simulink model "FrameStructTest"  (R2022b)
settings: Solver=VariableStepAuto  StartTime=0.0  StopTime=0.01  RelTol=1e-3
model workspace (MAT data in the model file):
  f_s = Simulink.Parameter
  f_s.Value = 0.0001
  f_s.DataType = 'double'
  f_s.Complexity = 'real'
  f_s.Dimensions = [1 1]
libraries: simulink x24, hdlsllib x14, dspsigops x8, commdigbbndapm x3, dsphdlfiltering2 x2, commfilt2 x2, commdigbbndpm3 x2, commrandsrc3 x1
(part 1 of 2)
settings Model: Creator=svdvl  LastModifiedBy=User

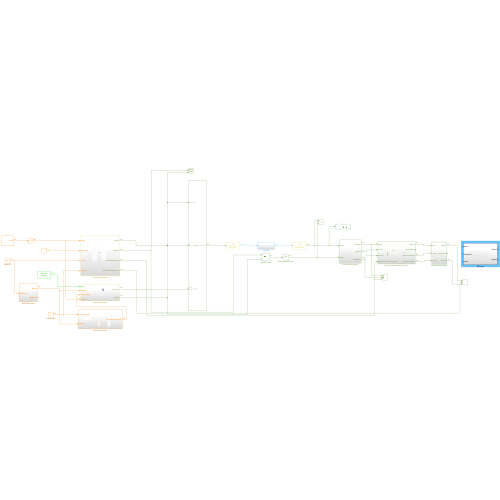
[thumbnail: Simulink's stored preview of the top-level diagram]
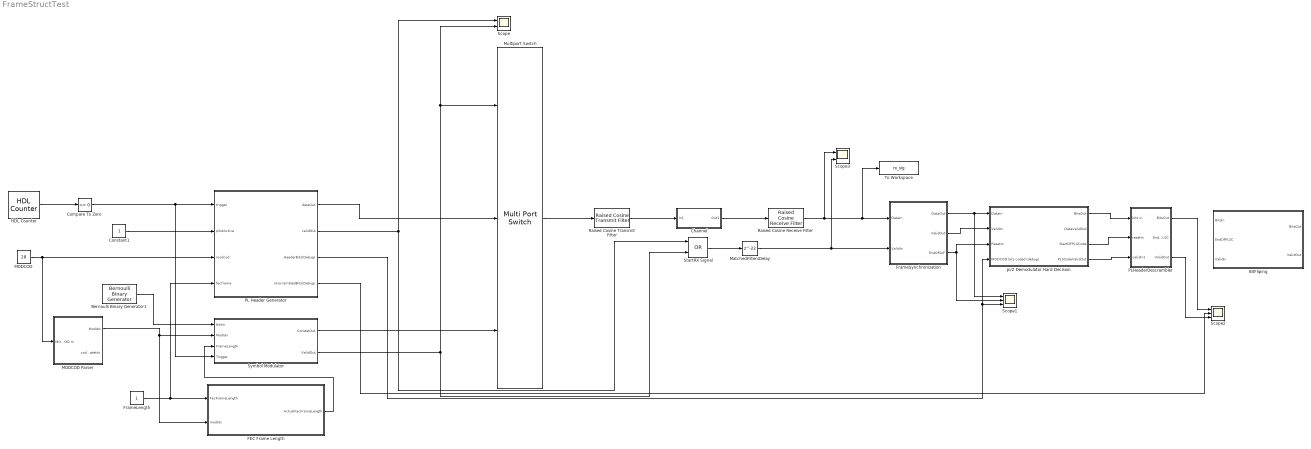
== system FrameStructTest ==
  Bernoulli Binary Generator1 : commrandsrc3/Bernoulli Binary Generator  ProbabilityOfZero=0.5  SeedSource=Auto  Seed=0  SampleTime=f_s/32*7/10  SamplesPerFrame=1  OutputDataType=uint8  SimulateUsing=Code generation
  BitFliping : Subsystem
  Channel : Subsystem
  Compare To Zero : simulink/Logic and Bit Operations/Compare To Zero  relop===  OutDataTypeStr=boolean
  Constant1 : Constant  SampleTime=f_s
  FEC Frame Length : Subsystem
  FrameLength : Constant  SampleTime=f_s
  FrameSynchronization : Subsystem
  HDL Counter : hdlsllib/Sources/HDL Counter  CountType=Count limited  CountInit=0  CountStep=1  CountMax=12960  CountFromType=Initial value  CountFrom=0  CountResetPort=off  CountLoadPort=off  CountEnbPort=off  CountDirPort=off  CountHitOutputPort=off  CountDataType=Unsigned  CountWordLen=14  CountFracLen=0  CountSampTime=f_s
  MODCOD : Constant  Value=28  VectorParams1D=off  OutDataTypeStr=uint8  SampleTime=f_s
  MODCOD Parser : Subsystem
  MatchedFiltersDelay : Delay  DelayLength=22
  Multiport Switch : MultiPortSwitch  DataPortOrder=Zero-based contiguous  Inputs=2  zeroidx=on  SaturateOnIntegerOverflow=off  InputSameDT=off
  PL Header Generator : Subsystem
  PLHeaderDescrambler : Subsystem
  Raised Cosine Receive Filter : commfilt2/Raised Cosine Receive Filter  filtType=Square root  R=0.2  filtSpan=20  N=2  downFactor=2  downOffset=0  filterGain=1  RateOptions=Allow multirate processing  framing=Mute  checkCoeff=off  variableName=rcRxFilt  currentFiltSpan=10  D=5  inputOffset=0  sampMode=Mute  saveAsFlag=0  rateMode=Downsampling  checkGain=Normalized  launchFVT=on  roundingMode=Floor  overflowMode=off  coeffDataTypeStr=Inherit: Same word length as input  coeffMin=[]  coeffMax=[]  coeffLastDataTypeStr=Inherit: Same word length as input  accumDataTypeStr=Inherit: Same as product output  accumLastDataTypeStr=Inherit: Same as product output  outputDataTypeStr=Inherit: Same as accumulator  outputMin=[]  outputMax=[]  outputLastDataTypeStr=Inherit: Same as accumulator
      settings: LibrarySourceBlock=|
      | commhdlfilt/Raised Cosine
      | Receive Filter
  Raised Cosine Transmit Filter : commfilt2/Raised Cosine Transmit Filter  filtType=Square root  R=0.2  filtSpan=20  N=2  filterGain=1  RateOptions=Allow multirate processing  framing=Mute  checkCoeff=off  variableName=rcTxFilt  checkGain=Normalized  sampMode=Mute  saveAsFlag=0  currentFiltSpan=10  D=5  launchFVT=on  roundingMode=Floor  overflowMode=off  coeffDataTypeStr=Inherit: Same word length as input  coeffMin=[]  coeffMax=[]  coeffLastDataTypeStr=Inherit: Same word length as input  outputDataTypeStr=Inherit: Same as accumulator  outputMin=[]  outputMax=[]  outputLastDataTypeStr=Inherit: Same as accumulator
      settings: LibrarySourceBlock=|
      | commhdlfilt/Raised Cosine
      | Transmit Filter
  Scope : Scope  NumInputPorts=2
  Scope1 : Scope  NumInputPorts=3
  Scope2 : Scope  NumInputPorts=3
  Scope3 : Scope  NumInputPorts=2
  StartRX Signal : Logic  Operator=OR  AllPortsSameDT=off  OutDataTypeStr=boolean
  Symbol Modulator : Subsystem
  To Workspace : ToWorkspace  VariableName=rx_sig  SampleTime=-1
      settings: Save2DSignal=2-D array (concatenate along first dimension)
  pi/2 Demodulator Hard Decision : Subsystem
  wires:
  HDL Counter/1 -> Compare To Zero/1
  FEC Frame Length/1(ActualFecFrameLength) -> Symbol Modulator/3(FrameLength)
  MODCOD Parser/1(ModIdx) -> FEC Frame Length/2(modIdx), Symbol Modulator/2(ModIdx)
  Bernoulli Binary Generator1/1 -> Symbol Modulator/1(bitsIn)
  Symbol Modulator/1(ConstelOut) -> Multiport Switch/3
  MODCOD/1 -> PL Header Generator/3(modcod), MODCOD Parser/1(MODCOD In)
  FrameLength/1 -> PL Header Generator/4(fecframe), FEC Frame Length/1(FecFrameLength)
  Compare To Zero/1 -> PL Header Generator/1(trigger), Symbol Modulator/4(Trigger)
  PL Header Generator/2(validOut) -> StartRX Signal/1, Scope/1
  Symbol Modulator/2(ValidOut) -> StartRX Signal/2, Multiport Switch/1, Scope/2
  PL Header Generator/1(dataOut) -> Multiport Switch/2
  Raised Cosine Transmit Filter/1 -> Channel/1(In1)
  Channel/1(Out1) -> Raised Cosine Receive Filter/1
  Raised Cosine Receive Filter/1 -> Scope3/1, To Workspace/1, FrameSynchronization/1(DataIn)
  Multiport Switch/1 -> Raised Cosine Transmit Filter/1
  FrameSynchronization/1(DataOut) -> Scope1/1, pi/2 Demodulator Hard Decision/1(DataIn)
  FrameSynchronization/2(ValidOut) -> pi/2 Demodulator Hard Decision/2(ValidIn)
  FrameSynchronization/3(EndOfSoF) -> Scope1/2, pi/2 Demodulator Hard Decision/3(ResetIn)
  PL Header Generator/3(HeaderBits(Debug)) -> Scope1/3, pi/2 Demodulator Hard Decision/4(MODCOD bits coded (debug))
  pi/2 Demodulator Hard Decision/1(BitsOut) -> PLHeaderDescrambler/1(bits in)
  pi/2 Demodulator Hard Decision/3(StartOFPLSCode) -> PLHeaderDescrambler/2(resetIn)
  pi/2 Demodulator Hard Decision/4(PLSCodeValidOut) -> PLHeaderDescrambler/3(validIn1)
  PLHeaderDescrambler/1(BitsOut) -> Scope2/1
  PL Header Generator/4(UnscrambledBits(Debug)) -> Scope2/2
  PLHeaderDescrambler/3(ValidOut) -> Scope2/3
  Constant1/1 -> PL Header Generator/2(pilotActive)
  StartRX Signal/1 -> MatchedFiltersDelay/1
  MatchedFiltersDelay/1 -> Scope3/2, FrameSynchronization/2(ValidIn)

== system FrameStructTest/BitFliping ==
  note: Bit 7 at the output
  BitsIn : Inport
  EndOfPLSC : Inport  Port=2
  ValidIn : Inport  Port=3
  Delay : Delay  DelayLength=1
  Delay1 : Delay  DelayLength=1
  Enabled Delay : Delay  DelayLength=1  ShowEnablePort=on
      settings: InputPortMap=u0,e6
  HDL Counter : hdlsllib/Sources/HDL Counter  CountType=Count limited  CountInit=0  CountStep=1  CountMax=1  CountFromType=Initial value  CountFrom=0  CountResetPort=off  CountLoadPort=off  CountEnbPort=on  CountDirPort=off  CountHitOutputPort=off  CountDataType=Unsigned  CountWordLen=8  CountFracLen=0  CountSampTime=1
  Logical Operator : Logic  Operator=XOR  AllPortsSameDT=off  OutDataTypeStr=boolean
  Logical Operator1 : Logic  Operator=NOT  AllPortsSameDT=off  OutDataTypeStr=boolean
  Switch : Switch  Criteria=u2 > Threshold  SaturateOnIntegerOverflow=off  InputSameDT=off
  Switch1 : Switch  Criteria=u2 ~= 0  SaturateOnIntegerOverflow=off  InputSameDT=off
  BitsOut : Outport
  ValidOut : Outport  Port=2
  wires:
  BitsIn/1 -> Delay/1, Logical Operator1/1, Delay1/1, Switch/1, Logical Operator/1
  Delay/1 -> Logical Operator/2
  Switch1/1 -> BitsOut/1
  ValidIn/1 -> HDL Counter/1
  HDL Counter/1 -> Enabled Delay/2, Switch/2
  Logical Operator/1 -> Enabled Delay/1
  Enabled Delay/1 -> Switch1/2
  Logical Operator1/1 -> Switch/3
  Switch/1 -> Switch1/3
  Delay1/1 -> Switch1/1

== system FrameStructTest/Channel ==
  In1 : Inport
  Out1 : Outport
  wires:
  In1/1 -> Out1/1

== system FrameStructTest/FEC Frame Length ==
  note: modIdx encodes the number of bits in a symbol
      | 0 -- 2 bits per constellation point
      | 1 -- 3 bits
      | 2 -- 4 bits
      | 3 -- 5 bits
      | 4 -- 6 bits
  note: 0 normal frame
      | 1 short frame
      | 2 medium frame
  note: number of symbols in FEC Frame
  FecFrameLength : Inport
  modIdx : Inport  Port=2
  Medium Frame xFECFrame Length1 : Lookup_n-D  NumberOfTableDimensions=1  BreakpointsSpecification=Even spacing  BreakpointsForDimension1=[-5:5]  BreakpointsForDimension1FirstPoint=0  Table=32400./log2([4 8 16 32 64])  TableDataTypeStr=fixdt(0,15,0)  InterpMethod=Flat  InternalRulePriority=Speed  OutDataTypeStr=fixdt(0,15,0)  RndMeth=Simplest
  Multiport Switch : MultiPortSwitch  SaturateOnIntegerOverflow=off  InputSameDT=off
  Normal Frame xFECFrame Length : Lookup_n-D  NumberOfTableDimensions=1  BreakpointsSpecification=Even spacing  BreakpointsForDimension1=[-5:5]  BreakpointsForDimension1FirstPoint=0  Table=64800./log2([4 8 16 32 64])  TableDataTypeStr=fixdt(0,15,0)  InterpMethod=Flat  InternalRulePriority=Speed  OutDataTypeStr=fixdt(0,15,0)  RndMeth=Simplest
  Short Frame xFECFrame Length : Lookup_n-D  NumberOfTableDimensions=1  BreakpointsSpecification=Even spacing  BreakpointsForDimension1=[-5:5]  BreakpointsForDimension1FirstPoint=0  Table=16200./log2([4 8 16 32 64])  TableDataTypeStr=fixdt(0,15,0)  InterpMethod=Flat  InternalRulePriority=Speed  OutDataTypeStr=fixdt(0,15,0)  RndMeth=Simplest
  ActualFecFrameLength : Outport
  wires:
  Multiport Switch/1 -> ActualFecFrameLength/1
  modIdx/1 -> Medium Frame xFECFrame Length1/1, Short Frame xFECFrame Length/1, Normal Frame xFECFrame Length/1
  FecFrameLength/1 -> Multiport Switch/1
  Medium Frame xFECFrame Length1/1 -> Multiport Switch/4
  Short Frame xFECFrame Length/1 -> Multiport Switch/3
  Normal Frame xFECFrame Length/1 -> Multiport Switch/2

== system FrameStructTest/FrameSynchronization ==
  DataIn : Inport
  ValidIn : Inport  Port=2
  Correlator : Subsystem
  Delay : Delay  DelayLength=70
  Delay1 : Delay  DelayLength=70
  Delay2 : Delay  DelayLength=44
  Delay3 : Delay  DelayLength=44
  Peak Detector : Subsystem
  DataOut : Outport
  ValidOut : Outport  Port=2
  EndOfSoF : Outport  Port=3
  wires:
  DataIn/1 -> Correlator/1(DataIn), Delay/1
  ValidIn/1 -> Correlator/2(ValidIn), Delay1/1
  Peak Detector/1(thersholdExceeded) -> EndOfSoF/1
  Correlator/1(SoFCorrelator) -> Peak Detector/1(SOFCorr)
  Correlator/2(PLSCCorrelator) -> Peak Detector/2(PLSCCorr)
  Correlator/3(Threshold) -> Peak Detector/3(threshold)
  Delay/1 -> Delay2/1
  Delay1/1 -> Delay3/1
  Delay2/1 -> DataOut/1
  Delay3/1 -> ValidOut/1

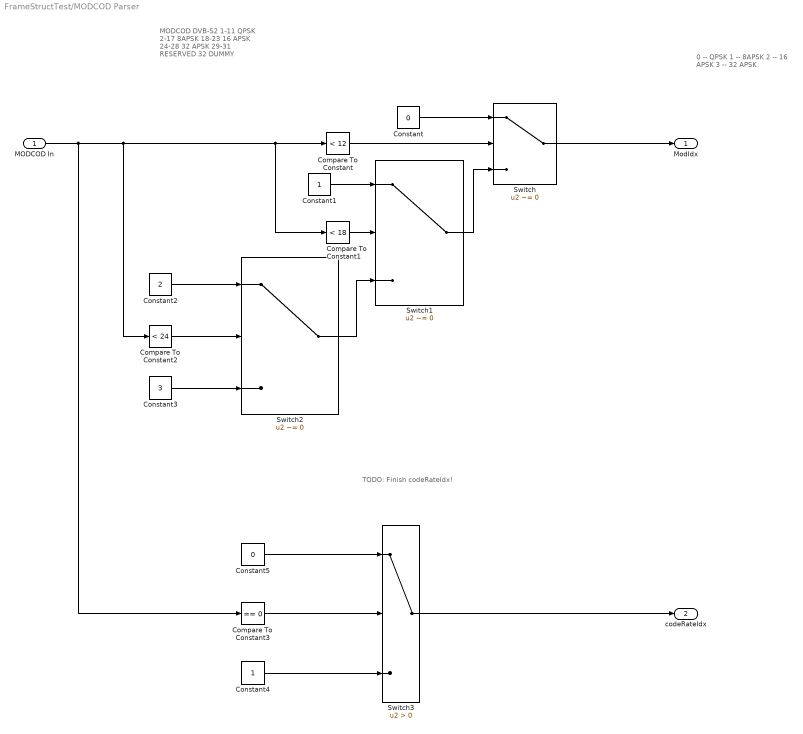
== system FrameStructTest/MODCOD Parser ==
  note: TODO: Finish codeRateIdx!
  note: MODCOD DVB-S2
      | 1-11 QPSK
      | 2-17 8APSK
      | 18-23 16 APSK
      | 24-28 32 APSK
      | 29-31 RESERVED
      | 32 DUMMY
  note: 0 -- QPSK
      | 1 -- 8APSK
      | 2 -- 16 APSK
      | 3 -- 32 APSK
  MODCOD In : Inport
  Compare To Constant : simulink/Logic and Bit Operations/Compare To Constant  relop=<  const=12  OutDataTypeStr=boolean
  Compare To Constant1 : simulink/Logic and Bit Operations/Compare To Constant  relop=<  const=18  OutDataTypeStr=boolean
  Compare To Constant2 : simulink/Logic and Bit Operations/Compare To Constant  relop=<  const=24  OutDataTypeStr=boolean
  Compare To Constant3 : simulink/Logic and Bit Operations/Compare To Constant  relop===  const=0  OutDataTypeStr=boolean
  Constant : Constant  Value=0  SampleTime=f_s
  Constant1 : Constant  SampleTime=f_s
  Constant2 : Constant  Value=2  SampleTime=f_s
  Constant3 : Constant  Value=3  SampleTime=f_s
  Constant4 : Constant  SampleTime=-1
  Constant5 : Constant  Value=0  SampleTime=-1
  Switch : Switch  Criteria=u2 ~= 0  SaturateOnIntegerOverflow=off  InputSameDT=off
  Switch1 : Switch  Criteria=u2 ~= 0  SaturateOnIntegerOverflow=off  InputSameDT=off
  Switch2 : Switch  Criteria=u2 ~= 0  SaturateOnIntegerOverflow=off  InputSameDT=off
  Switch3 : Switch  Criteria=u2 > Threshold  SaturateOnIntegerOverflow=off  InputSameDT=off
  ModIdx : Outport
  codeRateIdx : Outport  Port=2
  wires:
  MODCOD In/1 -> Compare To Constant3/1, Compare To Constant1/1, Compare To Constant/1, Compare To Constant2/1
  Switch/1 -> ModIdx/1
  Compare To Constant/1 -> Switch/2
  Constant/1 -> Switch/1
  Switch1/1 -> Switch/3
  Compare To Constant1/1 -> Switch1/2
  Constant1/1 -> Switch1/1
  Switch2/1 -> Switch1/3
  Compare To Constant2/1 -> Switch2/2
  Constant2/1 -> Switch2/1
  Constant3/1 -> Switch2/3
  Switch3/1 -> codeRateIdx/1
  Compare To Constant3/1 -> Switch3/2
  Constant5/1 -> Switch3/1
  Constant4/1 -> Switch3/3

== system FrameStructTest/PL Header Generator ==
  note: 1 at the start of the frame, else zero
  trigger : Inport
  pilotActive : Inport  Port=2
  modcod : Inport  Port=3
  fecframe : Inport  Port=4
  PL Header Bits Generator : Subsystem
  Scope : Scope  NumInputPorts=2
  Terminator : Terminator
  pi2 BSPK Modulator : Subsystem
  dataOut : Outport
  validOut : Outport  Port=2
  HeaderBits(Debug) : Outport  Port=3
  UnscrambledBits(Debug) : Outport  Port=4
  wires:
  PL Header Bits Generator/1(bitsOut) -> HeaderBits(Debug)/1, pi2 BSPK Modulator/1(bitsIn)
  PL Header Bits Generator/2(bitsStart) -> pi2 BSPK Modulator/2(startIn)
  PL Header Bits Generator/4(bitsValid) -> pi2 BSPK Modulator/3(validIn)
  PL Header Bits Generator/3(bitsEnd) -> Terminator/1
  trigger/1 -> PL Header Bits Generator/1(trigger)
  pilotActive/1 -> PL Header Bits Generator/2(pilotActive)
  modcod/1 -> PL Header Bits Generator/3(modcod)
  fecframe/1 -> PL Header Bits Generator/4(fecframe)
  pi2 BSPK Modulator/2(validOut) -> Scope/2, validOut/1
  PL Header Bits Generator/5(UnscrambledBits) -> UnscrambledBits(Debug)/1
  pi2 BSPK Modulator/1(dataOut) -> Scope/1, dataOut/1

== system FrameStructTest/PLHeaderDescrambler ==
  bits in : Inport
  resetIn : Inport  Port=2
  validIn1 : Inport  Port=3
  1-D Lookup Table : Lookup_n-D  NumberOfTableDimensions=1  LookupTableObject=''  BreakpointsSpecification=Even spacing  BreakpointsForDimension1=[-5:5]  BreakpointsForDimension1FirstPoint=0  BreakpointsForDimension2FirstPoint=10  BreakpointsForDimension2Spacing=12  IndexSearchMethod=Evenly spaced points  Table=[1 0 1 1 1 1 0 0 0 0 0 1 0 0 0 1 1 0 0 0 0 0 0 0 1 0 1 0 0 1 0 1 0 1 0 1 0 0 0 1 0 1 1 1 0 1 1 1 0 1 0 1 1 1 0 0 1 0 0 1 1 1 0 1 1 0 0 0 0 1 0 1 1 0 0 0 1 1 1 1 1 1 0 1 1 0 1 0 1 1 0 0 1 1 0 1 1 0 1 1 1 0 0 0 0 1 1 1 0 0 0 1 1 0 1 0 1 0 0 1 1 1 1 1 0 0 0 1 0 0 0 0 1 1 0 0 1 0 1 0 0 0 0 0 0 1 1 1 1 0 1 1 1 1]  InterpMethod=Flat  DiagnosticForOutOfRangeInput=Error  InternalRulePriority=Speed  RndMeth=Simplest
  Compare To Constant : simulink/Logic and Bit Operations/Compare To Constant  relop===  const=63  OutDataTypeStr=boolean
  Data Type Conversion : DataTypeConversion  OutDataTypeStr=boolean  SaturateOnIntegerOverflow=off  RndMeth=Floor
  Delay : Delay  DelayLength=1
  Delay1 : Delay  DelayLength=1
  Logical Operator : Logic  Operator=XOR  AllPortsSameDT=off  OutDataTypeStr=boolean
  Logical Operator1 : Logic  AllPortsSameDT=off  OutDataTypeStr=boolean
  PLSC Valid Counter : hdlsllib/Sources/HDL Counter  CountType=Count limited  CountInit=0  CountStep=1  CountMax=154-1  CountFromType=Initial value  CountFrom=0  CountResetPort=on  CountLoadPort=off  CountEnbPort=on  CountDirPort=off  CountHitOutputPort=off  CountDataType=Unsigned  CountWordLen=8  CountFracLen=0  CountSampTime=1
  Scope1 : Scope  NumInputPorts=2
  Scope2 : Scope  NumInputPorts=4
  BitsOut : Outport
  EndOfPLSC : Outport  Port=2
  ValidOut : Outport  Port=3
  wires:
  resetIn/1 -> Scope2/2, PLSC Valid Counter/1
  validIn1/1 -> Scope2/3, Delay/1, PLSC Valid Counter/2
  Delay/1 -> Logical Operator1/2, Scope1/2, ValidOut/1
  Logical Operator1/1 -> Scope1/1, EndOfPLSC/1
  bits in/1 -> Delay1/1
  Compare To Constant/1 -> Logical Operator1/1
  Data Type Conversion/1 -> Logical Operator/2
  PLSC Valid Counter/1 -> Compare To Constant/1, 1-D Lookup Table/1
  Logical Operator/1 -> Scope2/4, BitsOut/1
  1-D Lookup Table/1 -> Data Type Conversion/1
  Delay1/1 -> Scope2/1, Logical Operator/1

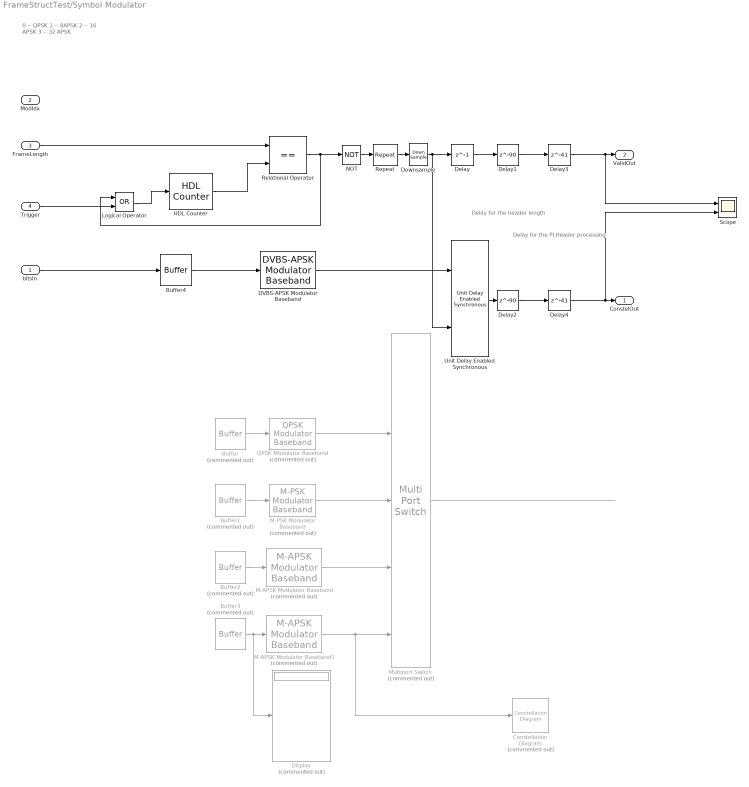
== system FrameStructTest/Symbol Modulator ==
  note: Delay for the PLHeader processing
  note: Delay for the header length
  note: 0 -- QPSK
      | 1 -- 8APSK
      | 2 -- 16 APSK
      | 3 -- 32 APSK
  bitsIn : Inport
  ModIdx : Inport  Port=2
  FrameLength : Inport  Port=3
  Trigger : Inport  Port=4
  Buffer : Buffer  Commented=on  N=2  OutputFrames=off
  Buffer1 : Buffer  Commented=on  N=3  OutputFrames=off
  Buffer2 : Buffer  Commented=on  N=4  OutputFrames=off
  Buffer3 : Buffer  Commented=on  N=5  OutputFrames=off
  Buffer4 : Buffer  N=5  OutputFrames=off
  Constellation Diagram : ConstellationDiagram  Commented=on  WindowPosition=[382.000000,84.000000,600.000000,600.000000,]  ScopeFrameLocation=window  DefaultConfigurationName=comm.scopes.ConstellationDiagramBlockCfg
  DVBS-APSK Modulator Baseband : commdigbbndapm/DVBS-APSK Modulator Baseband  StdSuffix=S2  FrameLength=Normal  ModOrder=32  CodeIDF=9/10  NormalizationMethod=Unit average power  InputType=Bit  OutputDataType=double  SimulateUsing=Code generation
      settings: LibrarySourceBlock=|
      | commdigbbndstd/DVBS-APSK
      | Modulator Baseband
  Delay : Delay  DelayLength=1
  Delay1 : Delay  DelayLength=90
  Delay2 : Delay  DelayLength=90
  Delay3 : Delay  DelayLength=41
  Delay4 : Delay  DelayLength=41
  Display : Display  Commented=on
  Downsample : DownSample  N=7  RateOptions=Allow multirate processing
  HDL Counter : hdlsllib/Sources/HDL Counter  CountType=Count limited  CountInit=1  CountStep=1  CountMax=64800  CountFromType=Initial value  CountFrom=1  CountResetPort=on  CountLoadPort=off  CountEnbPort=off  CountDirPort=off  CountHitOutputPort=off  CountDataType=Unsigned  CountWordLen=20  CountFracLen=0  CountSampTime=1
  Logical Operator : Logic  Operator=OR  AllPortsSameDT=off  OutDataTypeStr=boolean
  M-APSK Modulator Baseband : commdigbbndapm/M-APSK Modulator Baseband  Commented=on  ConstPointsCirclewise=[ 4, 12 ]  Radii=[ 0.5, 1 ]  PhaseOffset=[ pi/4, pi/12 ]  SymbolMapping=Auto  CustomSymbolMapping=[ 0, 4, 12, 8, 1, 3, 2, 6, 7, 5, 13, 15, 14, 10, 11, 9 ]  InputType=Bit  OutputDataType=double  SimulateUsing=Code generation
  M-APSK Modulator Baseband1 : commdigbbndapm/M-APSK Modulator Baseband  Commented=on  ConstPointsCirclewise=[ 4, 12, 16]  Radii=[ 0.5, 0.5*2.84, 0.5*5.27 ]  PhaseOffset=[ pi/4, pi/12, 0 ]  SymbolMapping=Auto  CustomSymbolMapping=[ 0, 4, 12, 8, 1, 3, 2, 6, 7, 5, 13, 15, 14, 10, 11, 9 ]  InputType=Bit  OutputDataType=double  SimulateUsing=Code generation
  M-PSK Modulator Baseband : commdigbbndpm3/M-PSK Modulator Baseband  Commented=on  M=8  InType=Bit  Enc=Gray  Mapping=[0:7]  Ph=0  outDtype=double  outWordLen=16  outUDDataType=sfix(16)  outFracLenMode=Best precision  outFracLen=15  outDataTypeStr=double  outLastDataTypeStr=double
  Multiport Switch : MultiPortSwitch  Commented=on  DataPortOrder=Zero-based contiguous  Inputs=4  zeroidx=on  SaturateOnIntegerOverflow=off  InputSameDT=off
  NOT : Logic  Operator=NOT  IconShape=distinctive  AllPortsSameDT=off  OutDataTypeStr=boolean
  QPSK Modulator Baseband : commdigbbndpm3/QPSK Modulator Baseband  Commented=on  InType=Bit  Enc=Gray  Ph=0  outDtype=double  outWordLen=16  outUDDataType=sfix(16)  outFracLenMode=Best precision  outFracLen=15  outDataTypeStr=double  outLastDataTypeStr=double
  Relational Operator : RelationalOperator  Operator===  OutDataTypeStr=boolean  RndMeth=Simplest  InputSameDT=off
  Repeat : dspsigops/Repeat  N=64  RateOptions=Allow multirate processing  ic=0  mode=Unused parameter value
      settings: LibrarySourceBlock=dsphdlsupportsigops/Repeat
  Scope : Scope  NumInputPorts=2
  Unit Delay Enabled Synchronous : hdlsllib/Discrete/Unit Delay Enabled Synchronous  InitialCondition=0.0  SampleTime=-1
  ConstelOut : Outport
  ValidOut : Outport  Port=2
  wires:
  M-APSK Modulator Baseband/1 -> Multiport Switch/4
  M-PSK Modulator Baseband/1 -> Multiport Switch/3
  ? -> Multiport Switch/1
  Buffer3/1 -> Display/1, M-APSK Modulator Baseband1/1
  Buffer2/1 -> M-APSK Modulator Baseband/1
  ? -> Buffer/1, Buffer3/1, Buffer2/1, Buffer1/1
  Multiport Switch/1 -> ?
  M-APSK Modulator Baseband1/1 -> Constellation Diagram/1, Multiport Switch/5
  Buffer/1 -> QPSK Modulator Baseband/1
  QPSK Modulator Baseband/1 -> Multiport Switch/2
  Buffer1/1 -> M-PSK Modulator Baseband/1
  bitsIn/1 -> Buffer4/1
  Buffer4/1 -> DVBS-APSK Modulator Baseband/1
  FrameLength/1 -> Relational Operator/1
  HDL Counter/1 -> Relational Operator/2
  Trigger/1 -> Logical Operator/2
  Logical Operator/1 -> HDL Counter/1
  Relational Operator/1 -> NOT/1, Logical Operator/1
  NOT/1 -> Repeat/1
  DVBS-APSK Modulator Baseband/1 -> Unit Delay Enabled Synchronous/1
  Unit Delay Enabled Synchronous/1 -> Delay2/1
  Delay/1 -> Delay1/1
  Delay1/1 -> Delay3/1
  Delay2/1 -> Delay4/1
  Repeat/1 -> Downsample/1
  Downsample/1 -> Unit Delay Enabled Synchronous/2, Delay/1
  Delay3/1 -> Scope/1, ValidOut/1
  Delay4/1 -> Scope/2, ConstelOut/1

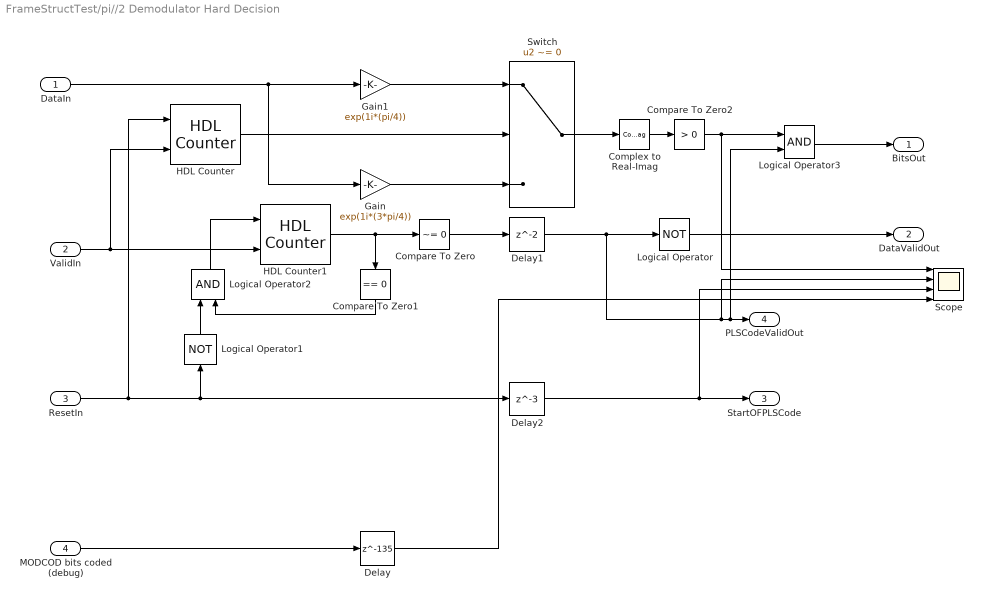
== system FrameStructTest/pi//2 Demodulator Hard Decision ==
  DataIn : Inport
  ValidIn : Inport  Port=2
  ResetIn : Inport  Port=3
  MODCOD bits coded (debug) : Inport  Port=4
  Compare To Zero : simulink/Logic and Bit Operations/Compare To Zero  relop=~=  OutDataTypeStr=boolean
  Compare To Zero1 : simulink/Logic and Bit Operations/Compare To Zero  relop===  OutDataTypeStr=boolean
  Compare To Zero2 : simulink/Logic and Bit Operations/Compare To Zero  relop=>  OutDataTypeStr=boolean
  Complex to Real-Imag : ComplexToRealImag  Output=Real
  Delay : Delay  DelayLength=135
  Delay1 : Delay
  Delay2 : Delay  DelayLength=3
  Gain : Gain  Gain=exp(1i*(3*pi/4))  ParamDataTypeStr=Inherit: Inherit from 'Gain'  OutDataTypeStr=Inherit: Same as input
  Gain1 : Gain  Gain=exp(1i*(pi/4))  ParamDataTypeStr=Inherit: Inherit from 'Gain'  OutDataTypeStr=Inherit: Same as input
  HDL Counter : hdlsllib/Sources/HDL Counter  CountType=Count limited  CountInit=0  CountStep=1  CountMax=1  CountFromType=Initial value  CountFrom=0  CountResetPort=on  CountLoadPort=off  CountEnbPort=on  CountDirPort=off  CountHitOutputPort=off  CountDataType=Unsigned  CountWordLen=8  CountFracLen=0  CountSampTime=1
  HDL Counter1 : hdlsllib/Sources/HDL Counter  CountType=Count limited  CountInit=0  CountStep=1  CountMax=64  CountFromType=Initial value  CountFrom=0  CountResetPort=on  CountLoadPort=off  CountEnbPort=on  CountDirPort=off  CountHitOutputPort=off  CountDataType=Unsigned  CountWordLen=8  CountFracLen=0  CountSampTime=1
  Logical Operator : Logic  Operator=NOT  AllPortsSameDT=off  OutDataTypeStr=boolean
  Logical Operator1 : Logic  Operator=NOT  AllPortsSameDT=off  OutDataTypeStr=boolean
  Logical Operator2 : Logic  AllPortsSameDT=off  OutDataTypeStr=boolean
  Logical Operator3 : Logic  AllPortsSameDT=off  OutDataTypeStr=boolean
  Scope : Scope  NumInputPorts=4
  Switch : Switch  Criteria=u2 ~= 0  SaturateOnIntegerOverflow=off  InputSameDT=off
  BitsOut : Outport
  DataValidOut : Outport  Port=2
  StartOFPLSCode : Outport  Port=3
  PLSCodeValidOut : Outport  Port=4
  wires:
  ResetIn/1 -> Logical Operator1/1, Delay2/1, HDL Counter/1
  ValidIn/1 -> HDL Counter1/2, HDL Counter/2
  HDL Counter/1 -> Switch/2
  DataIn/1 -> Gain1/1, Gain/1
  Gain1/1 -> Switch/1
  Gain/1 -> Switch/3
  HDL Counter1/1 -> Compare To Zero1/1, Compare To Zero/1
  Compare To Zero/1 -> Delay1/1
  Logical Operator/1 -> DataValidOut/1
  Logical Operator1/1 -> Logical Operator2/1
  Compare To Zero1/1 -> Logical Operator2/2
  Logical Operator2/1 -> HDL Counter1/1
  MODCOD bits coded (debug)/1 -> Delay/1
  Delay/1 -> Scope/4
  Delay1/1 -> Logical Operator/1, Scope/2, Logical Operator3/2, PLSCodeValidOut/1
  Delay2/1 -> Scope/3, StartOFPLSCode/1
  Switch/1 -> Complex to Real-Imag/1
  Complex to Real-Imag/1 -> Compare To Zero2/1
  Compare To Zero2/1 -> Logical Operator3/1, Scope/1
  Logical Operator3/1 -> BitsOut/1

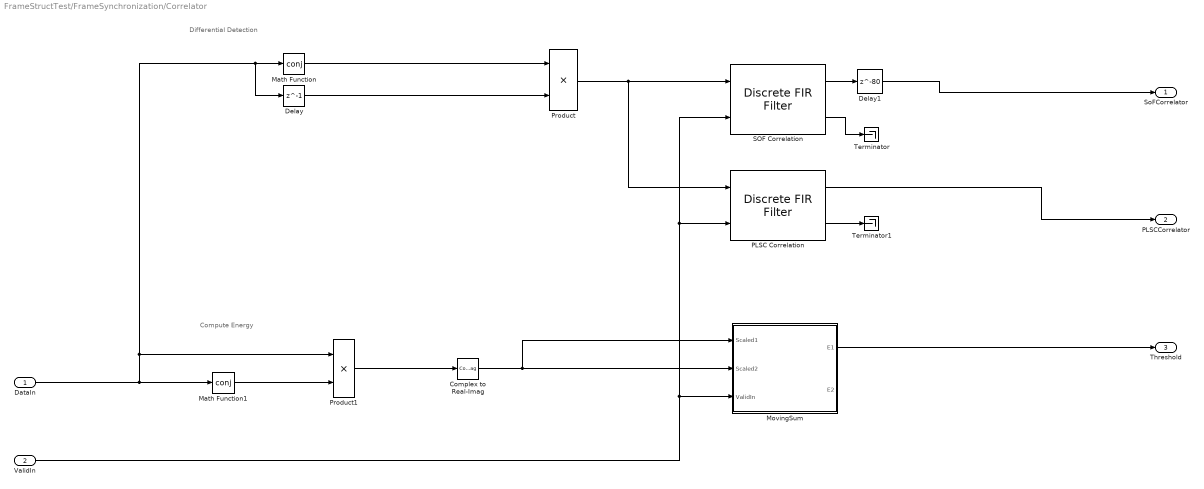
== system FrameStructTest/FrameSynchronization/Correlator ==
  note: Differential Detection
  note: Compute Energy
  DataIn : Inport
  ValidIn : Inport  Port=2
  Complex to Real-Imag : ComplexToRealImag  Output=Real
  Delay : Delay  DelayLength=1
  Delay1 : Delay  DelayLength=80
  Math Function : Math  Operator=conj
  Math Function1 : Math  Operator=conj
  MovingSum : Subsystem
  PLSC Correlation : dsphdlfiltering2/Discrete FIR Filter  NumeratorSource=Property  Numerator="flip([0.00207587049212865 + 1.00237167975181i\t0.00000000000000 + 0.00000000000000i\t8.97841895338702e-05 + 1.00037166900777i\t0.00000000000000 + 0.00000000000000i\t-0.00150009862867717 - 1.00261172640641i\t0.00000000000000 + 0.00000000000000i\t-0.00186313527990301 + 0.996924303079438i\t0.00000000000000 + 0.00000000000000i\t-0.00176874510379926 - 0.998123746787447i\t0.00000000000000 + 0.00000000000000i\t0.00351825220295110 + 1.00243783464914i\t0.00000000000000 + 0.00000000000000i\t-0.00104923899487630 - 1.00212768647515i\t0.00000000000000 + 0.00000000000000i\t-9.08941366732918e-05 - 1.00279065976558i\t0.00000000000000 + 0.00000000000000i\t0.000264511267563772 + 0.994765012470802i\t0.00000000000000 + 0.00000000000000i\t-0.000354605101616778 + 0.998050063639308i\t0.00000000000000 + 0.00000000000000i\t-0.00156509993050963 - 1.00006401581498i\t0.00000000000000 + 0.00000000000000i\t-0.00379695600052438 - 1.00139885511569i\t0.00000000000000 + 0.00000000000000i\t0.000329023206098233 + 0.998352317884963i\t0.00000000000000 + 0.00000000000000i\t-0.000590902774422253 + 0.996840422969325i\t0.00000000000000 + 0.00000000000000i\t-0.00201336103373989 + 0.997462644900221i\t0.00000000000000 + 0.00000000000000i\t0.00118723852207253 + 0.997333792740890i\t0.00000000000000 + 0.00000000000000i\t-4.97899868873164e-06 - 0.997812309870580i\t0.00000000000000 + 0.00000000000000i\t0.00175276419797504 + 0.995284147275562i\t0.00000000000000 + 0.00000000000000i\t-0.00125204909784643 - 0.998480183830676i\t0.00000000000000 + 0.00000000000000i\t-0.000156161848597181 - 0.997875878331027i\t0.00000000000000 + 0.00000000000000i\t0.000915582181836960 + 0.997441223785563i\t0.00000000000000 + 0.00000000000000i\t-0.000714473378005121 + 0.999023750181081i\t0.00000000000000 + 0.00000000000000i\t0.000742692725197169 + 0.996640040451418i\t0.00000000000000 + 0.00000000000000i\t-0.000255762430226181 - 1.00071546328831i\t0.00000000000000 + 0.00000000000000i\t-0.00237644629731570 - 0.998103512910141i\t0.00000000000000 + 0.00000000000000i\t-0.00199897288585371 - 0.998207363125413i\t0.00000000000000 + 0.00000000000000i\t0.00106046474807930 - 0.997353689041293i\t0.00000000000000 + 0.00000000000000i\t-0.00196123730769182 - 1.00018118069824i\t0.00000000000000 + 0.00000000000000i\t0.00200702791234686 - 1.00022265537262i\t0.00000000000000 + 0.00000000000000i\t0.000303066330948121 + 1.00171302805839i\t0.00000000000000 + 0.00000000000000i\t-0.000858127766466321 - 0.996081051766369i\t0.00000000000000 + 0.00000000000000i\t-0.000574946392339404 - 0.996112866352626i])"  NumeratorPrototype=[]  FilterStructure=Direct form systolic  SerializationOption=Minimum number of cycles between valid input samples  NumCycles=2  NumberOfMultipliers=2  SimulateUsing=Code generation  roundingMode=Floor  overflowMode=off  CoefficientsDataTypeStr=Inherit: Same word length as input  ResetInputPort=off  HDLGlobalReset=off
  Product : Product  OutDataTypeStr=Inherit: Same as first input
  Product1 : Product  OutDataTypeStr=Inherit: Same as first input
  SOF Correlation : dsphdlfiltering2/Discrete FIR Filter  NumeratorSource=Property  Numerator=flip([0.0000 - 1.0000i 0.0000 - 1.0000i 0.0000 - 1.0000i 0.0000 - 1.0000i 0.0000 + 1.0000i 0.0000 + 1.0000i 0.0000 + 1.0000i 0.0000 + 1.0000i 0.0000 - 1.0000i 0.0000 + 1.0000i 0.0000 + 1.0000i 0.0000 + 1.0000i 0.0000 - 1.0000i 0.0000 + 1.0000i 0.0000 + 1.0000i 0.0000 - 1.0000i 0.0000 - 1.0000i 0.0000 + 1.0000i 0.0000 - 1.0000i 0.0000 - 1.0000i 0.0000 + 1.0000i 0.0000 - 1.0000i 0.0000 + 1.0000i 0.0000 + 1.0000i 0.0000 - 1.0000i])  NumeratorPrototype=[]  FilterStructure=Direct form systolic  SerializationOption=Minimum number of cycles between valid input samples  NumCycles=2  NumberOfMultipliers=2  SimulateUsing=Code generation  roundingMode=Floor  overflowMode=off  CoefficientsDataTypeStr=Inherit: Same word length as input  ResetInputPort=off  HDLGlobalReset=off
  Terminator : Terminator
  Terminator1 : Terminator
  SoFCorrelator : Outport
  PLSCCorrelator : Outport  Port=2
  Threshold : Outport  Port=3
  wires:
  Delay1/1 -> SoFCorrelator/1
  Product/1 -> PLSC Correlation/1, SOF Correlation/1
  ValidIn/1 -> PLSC Correlation/2, SOF Correlation/2, MovingSum/3(ValidIn)
  DataIn/1 -> Math Function/1, Delay/1, Product1/1, Math Function1/1
  Math Function1/1 -> Product1/2
  MovingSum/1(E1) -> Threshold/1
  PLSC Correlation/2 -> Terminator1/1
  Math Function/1 -> Product/1
  SOF Correlation/2 -> Terminator/1
  SOF Correlation/1 -> Delay1/1
  Product1/1 -> Complex to Real-Imag/1
  Delay/1 -> Product/2
  Complex to Real-Imag/1 -> MovingSum/1(Scaled1), MovingSum/2(Scaled2)
  PLSC Correlation/1 -> PLSCCorrelator/1

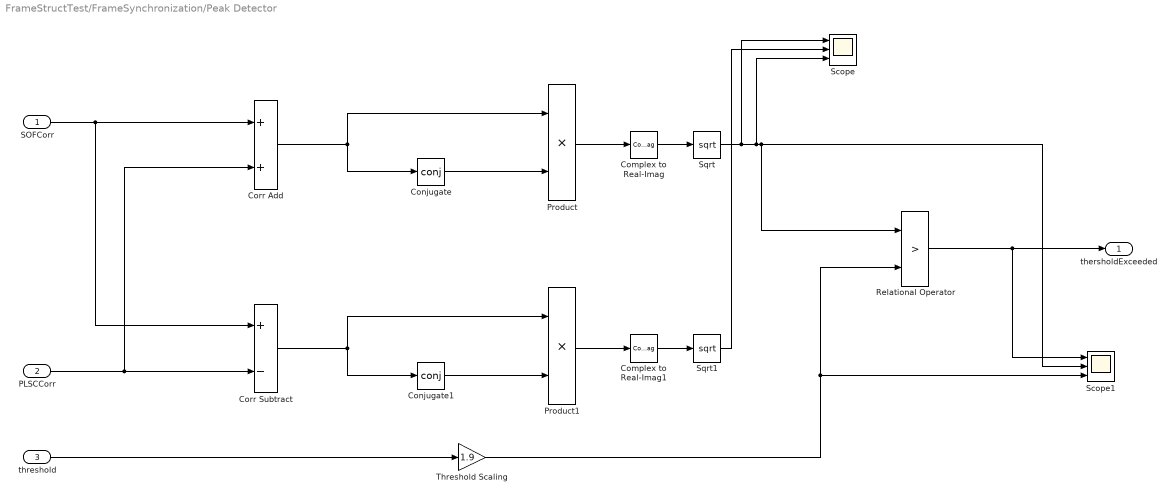
== system FrameStructTest/FrameSynchronization/Peak Detector ==
  SOFCorr : Inport
  PLSCCorr : Inport  Port=2
  threshold : Inport  Port=3
  Complex to Real-Imag : ComplexToRealImag  Output=Real
  Complex to Real-Imag1 : ComplexToRealImag  Output=Real
  Conjugate : Math  Operator=conj  SignedPower=on  RndMeth=Zero
  Conjugate1 : Math  Operator=conj  SignedPower=on  RndMeth=Zero
  Corr Add : Sum
  Corr Subtract : Sum  Inputs=+-
  Product : Product
  Product1 : Product
  Relational Operator : RelationalOperator  Operator=>  OutDataTypeStr=boolean  RndMeth=Simplest  InputSameDT=off
  Scope : Scope  NumInputPorts=3
  Scope1 : Scope  NumInputPorts=3
  Sqrt : Sqrt
  Sqrt1 : Sqrt
  Threshold Scaling : Gain  Gain=1.9  OutDataTypeStr=Inherit: Same as input
      mask init:
      | Simulink.suppressDiagnostic(gcb, 'SimulinkFixedPoint:util:fxpParameterPrecisionLoss');
  thersholdExceeded : Outport
  wires:
  PLSCCorr/1 -> Corr Add/2, Corr Subtract/2
  SOFCorr/1 -> Corr Subtract/1, Corr Add/1
  Corr Add/1 -> Product/1, Conjugate/1
  Conjugate/1 -> Product/2
  Product/1 -> Complex to Real-Imag/1
  Product1/1 -> Complex to Real-Imag1/1
  Conjugate1/1 -> Product1/2
  Corr Subtract/1 -> Product1/1, Conjugate1/1
  Complex to Real-Imag/1 -> Sqrt/1
  Complex to Real-Imag1/1 -> Sqrt1/1
  threshold/1 -> Threshold Scaling/1
  Sqrt/1 -> Scope/1, Scope/3, Scope1/2, Relational Operator/1
  Sqrt1/1 -> Scope/2
  Relational Operator/1 -> Scope1/1, thersholdExceeded/1
  Threshold Scaling/1 -> Scope1/3, Relational Operator/2

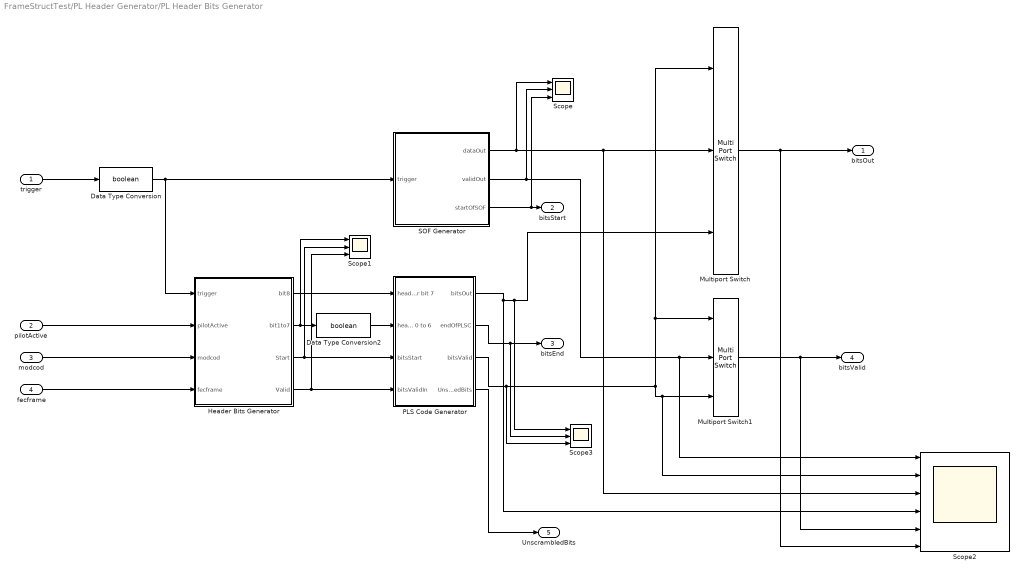
== system FrameStructTest/PL Header Generator/PL Header Bits Generator ==
  trigger : Inport
  pilotActive : Inport  Port=2
  modcod : Inport  Port=3
  fecframe : Inport  Port=4
  Data Type Conversion : DataTypeConversion  OutDataTypeStr=boolean  SaturateOnIntegerOverflow=off  RndMeth=Floor
  Data Type Conversion2 : DataTypeConversion  OutDataTypeStr=boolean  SaturateOnIntegerOverflow=off  RndMeth=Floor
  Header Bits Generator : Subsystem
  Multiport Switch : MultiPortSwitch  DataPortOrder=Zero-based contiguous  Inputs=2  zeroidx=on  SaturateOnIntegerOverflow=off  InputSameDT=off
  Multiport Switch1 : MultiPortSwitch  DataPortOrder=Zero-based contiguous  Inputs=2  zeroidx=on  SaturateOnIntegerOverflow=off  InputSameDT=off
  PLS Code Generator : Subsystem
  SOF Generator : Subsystem
  Scope : Scope  NumInputPorts=3
  Scope1 : Scope  NumInputPorts=3
  Scope2 : Scope  NumInputPorts=6
  Scope3 : Scope  NumInputPorts=3
  bitsOut : Outport
  bitsStart : Outport  Port=2
  bitsEnd : Outport  Port=3
  bitsValid : Outport  Port=4
  UnscrambledBits : Outport  Port=5
  wires:
  Data Type Conversion/1 -> Header Bits Generator/1(trigger), SOF Generator/1(trigger)
  SOF Generator/1(dataOut) -> Scope/1, Scope2/3, Multiport Switch/2
  PLS Code Generator/1(bitsOut) -> Scope2/4, Scope3/1, Multiport Switch/3
  PLS Code Generator/3(bitsValid) -> Scope3/3, Multiport Switch1/1, Multiport Switch/1, Scope2/2, Multiport Switch1/3
  Multiport Switch/1 -> Scope2/6, bitsOut/1
  SOF Generator/3(startOfSOF) -> Scope/3, bitsStart/1
  PLS Code Generator/2(endOfPLSC) -> Scope3/2, bitsEnd/1
  SOF Generator/2(validOut) -> Scope/2, Scope2/1, Multiport Switch1/2
  Multiport Switch1/1 -> Scope2/5, bitsValid/1
  trigger/1 -> Data Type Conversion/1
  pilotActive/1 -> Header Bits Generator/2(pilotActive)
  modcod/1 -> Header Bits Generator/3(modcod)
  fecframe/1 -> Header Bits Generator/4(fecframe)
  Header Bits Generator/2(bit1to7) -> Scope1/1, Data Type Conversion2/1
  Header Bits Generator/3(Start) -> PLS Code Generator/3(bitsStart), Scope1/2
  Header Bits Generator/4(Valid) -> PLS Code Generator/4(bitsValidIn), Scope1/3
  Header Bits Generator/1(bit8) -> PLS Code Generator/1(header bit 7)
  Data Type Conversion2/1 -> PLS Code Generator/2(header bits 0 to 6)
  PLS Code Generator/4(UnscrambledBits) -> UnscrambledBits/1

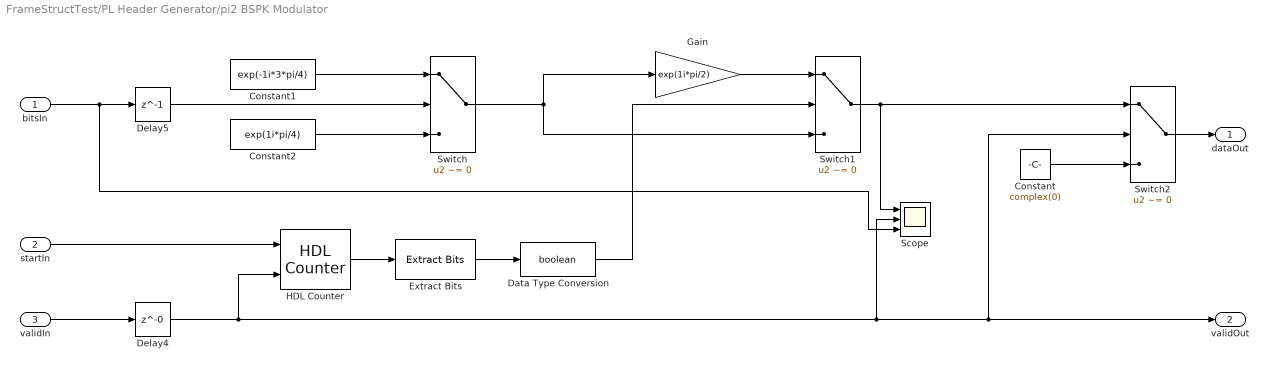
== system FrameStructTest/PL Header Generator/pi2 BSPK Modulator ==
  bitsIn : Inport
  startIn : Inport  Port=2
  validIn : Inport  Port=3
  Constant : Constant  Value=complex(0)  OutDataTypeStr=Inherit: Inherit via back propagation  SampleTime=-1
  Constant1 : Constant  Value=exp(-1i*3*pi/4)  OutDataTypeStr=double  SampleTime=-1
      mask init:
      | Simulink.suppressDiagnostic(gcb, 'SimulinkFixedPoint:util:fxpParameterPrecisionLoss');
  Constant2 : Constant  Value=exp(1i*pi/4)  OutDataTypeStr=double  SampleTime=-1
      mask init:
      | Simulink.suppressDiagnostic(gcb, 'SimulinkFixedPoint:util:fxpParameterPrecisionLoss');
  Data Type Conversion : DataTypeConversion  OutDataTypeStr=boolean  SaturateOnIntegerOverflow=off  RndMeth=Floor
  Delay4 : Delay  DelayLength=0
  Delay5 : Delay  DelayLength=1
  Extract Bits : simulink/Logic and Bit Operations/Extract Bits  bitsToExtract=Range of bits  numBits=8  bitIdxRange=0  outScalingMode=Treat bit field as an integer
  Gain : Gain  Gain=exp(1i*pi/2)  ParamDataTypeStr=fixdt(1,16,14)  OutDataTypeStr=Inherit: Same as input
      mask init:
      | Simulink.suppressDiagnostic(gcb, 'SimulinkFixedPoint:util:fxpParameterPrecisionLoss');
  HDL Counter : hdlsllib/Sources/HDL Counter  CountType=Count limited  CountInit=0  CountStep=1  CountMax=100  CountFromType=Initial value  CountFrom=0  CountResetPort=on  CountLoadPort=off  CountEnbPort=on  CountDirPort=off  CountHitOutputPort=off  CountDataType=Unsigned  CountWordLen=nextpow2(90 - 1)  CountFracLen=0  CountSampTime=1
  Scope : Scope  NumInputPorts=3
  Switch : Switch  Criteria=u2 ~= 0  SaturateOnIntegerOverflow=off  InputSameDT=off
  Switch1 : Switch  Criteria=u2 ~= 0  SaturateOnIntegerOverflow=off  InputSameDT=off
  Switch2 : Switch  Criteria=u2 ~= 0  SaturateOnIntegerOverflow=off  InputSameDT=off
  dataOut : Outport
  validOut : Outport  Port=2
  wires:
  Extract Bits/1 -> Data Type Conversion/1
  Gain/1 -> Switch1/1
  Delay4/1 -> HDL Counter/2, Switch2/2, validOut/1, Scope/2
  bitsIn/1 -> Scope/3, Delay5/1
  HDL Counter/1 -> Extract Bits/1
  validIn/1 -> Delay4/1
  startIn/1 -> HDL Counter/1
  Constant2/1 -> Switch/3
  Constant1/1 -> Switch/1
  Data Type Conversion/1 -> Switch1/2
  Delay5/1 -> Switch/2
  Switch/1 -> Switch1/3, Gain/1
  Switch1/1 -> Switch2/1, Scope/1
  Switch2/1 -> dataOut/1
  Constant/1 -> Switch2/3

== system FrameStructTest/FrameSynchronization/Correlator/MovingSum ==
  note: Delay by length of SoF sequence
  Scaled1 : Inport
  Scaled2 : Inport  Port=2
  ValidIn : Inport  Port=3
  Add : Sum  Inputs=|+-  OutDataTypeStr=Inherit: Same as first input
  Add1 : Sum  Inputs=|++  OutDataTypeStr=Inherit: Same as first input
  Add2 : Sum  Inputs=|+-  OutDataTypeStr=Inherit: Same as first input
  Add3 : Sum  Inputs=|++  OutDataTypeStr=Inherit: Same as first input
  Delay : Delay  DelayLength=26  ShowEnablePort=on
      settings: InputPortMap=u0,e6
  Delay1 : Delay  DelayLength=64  ShowEnablePort=on
      settings: InputPortMap=u0,e6
  Delay14 : Delay  DelayLength=1  ShowEnablePort=on
      settings: InputPortMap=u0,e6
  Delay2 : Delay  DelayLength=1  ShowEnablePort=on
      settings: InputPortMap=u0,e6
  E1 : Outport
  E2 : Outport  Port=2
  wires:
  Scaled1/1 -> Add/1, Delay/1
  Delay/1 -> Add/2
  Add/1 -> Add1/1
  Delay14/1 -> Add1/2
  Scaled2/1 -> Delay1/1, Add2/1
  Delay1/1 -> Add2/2
  ValidIn/1 -> Delay1/2, Delay/2, Delay14/2, Delay2/2
  Add2/1 -> Add3/1
  Delay2/1 -> Add3/2
  Add3/1 -> Delay2/1, E2/1
  Add1/1 -> E1/1, Delay14/1

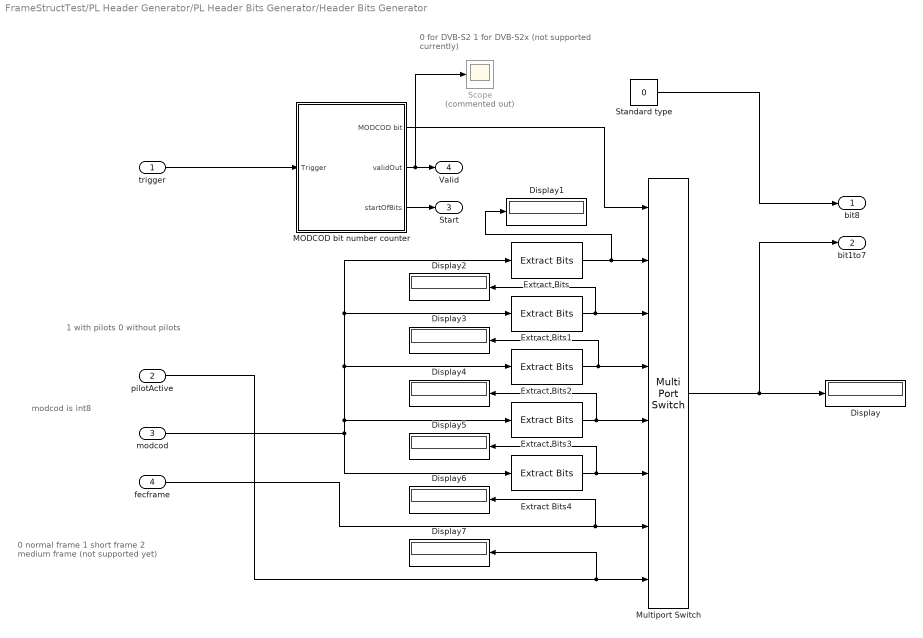
== system FrameStructTest/PL Header Generator/PL Header Bits Generator/Header Bits Generator ==
  note: modcod is int8
  note: 0 for DVB-S2
      | 1 for DVB-S2x (not supported currently)
  note: 1 with pilots
      | 0 without pilots
  note: 0 normal frame
      | 1 short frame
      | 2 medium frame (not supported yet)
  trigger : Inport
  pilotActive : Inport  Port=2
  modcod : Inport  Port=3
  fecframe : Inport  Port=4
  Display{,1..7} (8 alike) : Display
  Extract Bits : simulink/Logic and Bit Operations/Extract Bits  bitsToExtract=Range of bits  numBits=8  bitIdxRange=0  outScalingMode=Treat bit field as an integer
  Extract Bits1 : simulink/Logic and Bit Operations/Extract Bits  bitsToExtract=Range of bits  numBits=8  bitIdxRange=1  outScalingMode=Treat bit field as an integer
  Extract Bits2 : simulink/Logic and Bit Operations/Extract Bits  bitsToExtract=Range of bits  numBits=8  bitIdxRange=2  outScalingMode=Treat bit field as an integer
  Extract Bits3 : simulink/Logic and Bit Operations/Extract Bits  bitsToExtract=Range of bits  numBits=8  bitIdxRange=3  outScalingMode=Treat bit field as an integer
  Extract Bits4 : simulink/Logic and Bit Operations/Extract Bits  bitsToExtract=Range of bits  numBits=8  bitIdxRange=4  outScalingMode=Treat bit field as an integer
  MODCOD bit number counter : Subsystem
  Multiport Switch : MultiPortSwitch  DataPortOrder=Zero-based contiguous  Inputs=7  zeroidx=on  SaturateOnIntegerOverflow=off  InputSameDT=off
  Scope : Scope  Commented=on
  Standard type : Constant  Value=0  SampleTime=f_s/32*7
  bit8 : Outport
  bit1to7 : Outport  Port=2
  Start : Outport  Port=3
  Valid : Outport  Port=4
  wires:
  trigger/1 -> MODCOD bit number counter/1(Trigger)
  modcod/1 -> Extract Bits4/1, Extract Bits2/1, Extract Bits/1, Extract Bits1/1, Extract Bits3/1
  Extract Bits4/1 -> Display5/1, Multiport Switch/6
  Extract Bits3/1 -> Display4/1, Multiport Switch/5
  Extract Bits2/1 -> Display3/1, Multiport Switch/4
  Extract Bits1/1 -> Multiport Switch/3, Display2/1
  Extract Bits/1 -> Display1/1, Multiport Switch/2
  Multiport Switch/1 -> Display/1, bit1to7/1
  Standard type/1 -> bit8/1
  MODCOD bit number counter/3(startOfBits) -> Start/1
  MODCOD bit number counter/2(validOut) -> Scope/1, Valid/1
  fecframe/1 -> Display6/1, Multiport Switch/7
  MODCOD bit number counter/1(MODCOD bit) -> Multiport Switch/1
  pilotActive/1 -> Display7/1, Multiport Switch/8

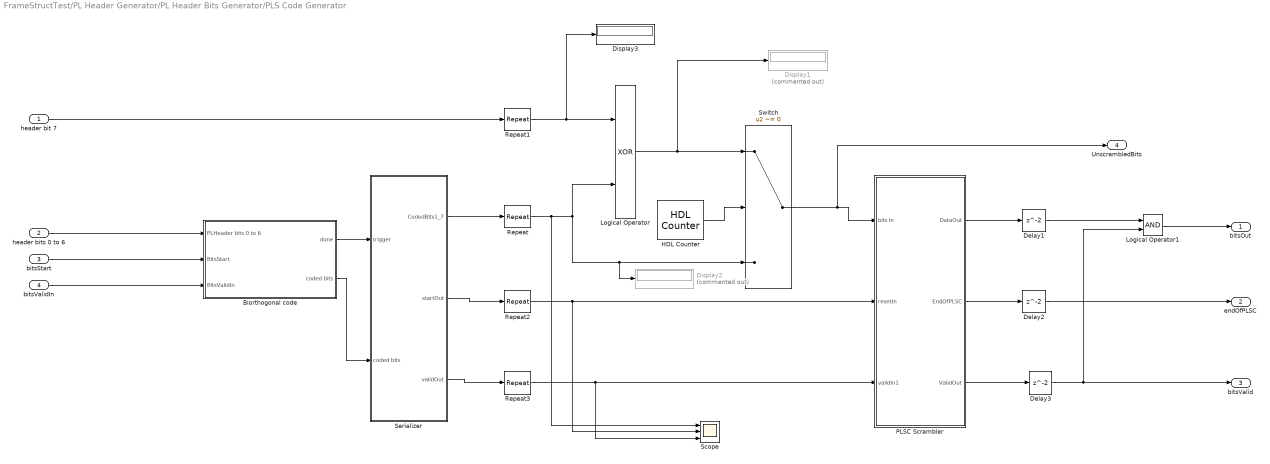
== system FrameStructTest/PL Header Generator/PL Header Bits Generator/PLS Code Generator ==
  header bit 7 : Inport
  header bits 0 to 6 : Inport  Port=2
  bitsStart : Inport  Port=3
  bitsValidIn : Inport  Port=4
  Biorthogonal code : Subsystem
  Delay1 : Delay
  Delay2 : Delay
  Delay3 : Delay
  Display1 : Display  Commented=on
  Display2 : Display  Commented=on
  Display3 : Display
  HDL Counter : hdlsllib/Sources/HDL Counter  CountType=Count limited  CountInit=0  CountStep=1  CountMax=1  CountFromType=Initial value  CountFrom=0  CountResetPort=off  CountLoadPort=off  CountEnbPort=off  CountDirPort=off  CountHitOutputPort=off  CountDataType=Unsigned  CountWordLen=1  CountFracLen=0  CountSampTime=-1
  Logical Operator : Logic  Operator=XOR  AllPortsSameDT=off  OutDataTypeStr=boolean
  Logical Operator1 : Logic  AllPortsSameDT=off  OutDataTypeStr=boolean
  PLSC Scrambler : Subsystem
  Repeat{,1..3} (4 alike) : dspsigops/Repeat  N=2  RateOptions=Allow multirate processing  ic=0  mode=Unused parameter value
  Scope : Scope  NumInputPorts=3
  Serializer : Subsystem
  Switch : Switch  Criteria=u2 ~= 0  SaturateOnIntegerOverflow=off  InputSameDT=off
  bitsOut : Outport
  endOfPLSC : Outport  Port=2
  bitsValid : Outport  Port=3
  UnscrambledBits : Outport  Port=4
  wires:
  header bits 0 to 6/1 -> Biorthogonal code/1(PLHeader bits 0 to 6)
  Serializer/1(CodedBits1_7) -> Repeat/1
  header bit 7/1 -> Repeat1/1
  Repeat/1 -> Scope/1, Switch/3, Display2/1, Logical Operator/2
  Repeat1/1 -> Display3/1, Logical Operator/1
  Logical Operator/1 -> Display1/1, Switch/1
  HDL Counter/1 -> Switch/2
  Switch/1 -> UnscrambledBits/1, PLSC Scrambler/1(bits in)
  PLSC Scrambler/1(DataOut) -> Delay1/1
  PLSC Scrambler/2(EndOfPLSC) -> Delay2/1
  PLSC Scrambler/3(ValidOut) -> Delay3/1
  bitsStart/1 -> Biorthogonal code/2(BitsStart)
  bitsValidIn/1 -> Biorthogonal code/3(BitsValidIn)
  Repeat2/1 -> Scope/2, PLSC Scrambler/2(resetIn)
  Serializer/2(startOut) -> Repeat2/1
  Serializer/3(validOut) -> Repeat3/1
  Repeat3/1 -> Scope/3, PLSC Scrambler/3(validIn1)
  Delay2/1 -> endOfPLSC/1
  Delay3/1 -> Logical Operator1/2, bitsValid/1
  Biorthogonal code/2(coded bits) -> Serializer/2(coded bits)
  Biorthogonal code/1(done) -> Serializer/1(trigger)
  Delay1/1 -> Logical Operator1/1
  Logical Operator1/1 -> bitsOut/1

== system FrameStructTest/PL Header Generator/PL Header Bits Generator/SOF Generator ==
  note: Compensating for the delay in PLSCODE generator
  note: 1 for the duration of SOF (25 samples)
  note: Outputs one when the first bit of SOF sequence is passed
  note: valid flag
      | 1 if output of subsystem is valid
      | 0 if invalid
  note: The SOF sequence bits
  note: Trigger that enables the SOF Generator
  note: Actual SOF values
  note: Counter limited to 25 (SOF length)
  trigger : Inport
  Data Type Conversion : DataTypeConversion  OutDataTypeStr=boolean  SaturateOnIntegerOverflow=off  RndMeth=Floor
  Delay : Delay  DelayLength=42
  Delay1 : Delay  DelayLength=42
  Delay2 : Delay  DelayLength=42
  Downsample : DownSample  N=7  RateOptions=Allow multirate processing
  Repeat : dspsigops/Repeat  N=32  InputProcessing=Columns as channels (frame based)  RateOptions=Allow multirate processing  ic=0  mode=Unused parameter value
      settings: LibrarySourceBlock=commsequence2/Repeat
  SOF Length Counter : Subsystem
  SOF Sequence : Lookup_n-D  NumberOfTableDimensions=1  BreakpointsSpecification=Even spacing  BreakpointsForDimension1=[-5:5]  BreakpointsForDimension1FirstPoint=0  Table=[0 1 1 0 0 0 1 1 0 1 0 0 1 0 1 1 1 0 1 0 0 0 0 0 1 0]  TableDataTypeStr=Inherit: Inherit from 'Table data'  InterpMethod=Flat  DiagnosticForOutOfRangeInput=Warning  InternalRulePriority=Speed  OutDataTypeStr=Inherit: Inherit from 'Table data'  RndMeth=Simplest
  Upsample : dspsigops/Upsample  N=2  phase=0  RateOptions=Allow multirate processing  ic=0  mode=Unused parameter value
  dataOut : Outport
  validOut : Outport  Port=2
  startOfSOF : Outport  Port=3
  wires:
  SOF Sequence/1 -> Data Type Conversion/1
  SOF Length Counter/1(LUT address) -> SOF Sequence/1
  Upsample/1 -> Repeat/1
  Data Type Conversion/1 -> Delay/1
  SOF Length Counter/2(validOut) -> Delay1/1
  SOF Length Counter/3(StartOfOSOF) -> Delay2/1
  trigger/1 -> Upsample/1
  Repeat/1 -> Downsample/1
  Downsample/1 -> SOF Length Counter/1(Trigger)
  Delay/1 -> dataOut/1
  Delay1/1 -> validOut/1
  Delay2/1 -> startOfSOF/1

== system FrameStructTest/PL Header Generator/PL Header Bits Generator/Header Bits Generator/MODCOD bit number counter ==
  Trigger : Inport
  Constant : Constant  SampleTime=f_s
  Data Type Conversion : DataTypeConversion  OutDataTypeStr=boolean  SaturateOnIntegerOverflow=off  RndMeth=Floor
  HDL Counter1 : hdlsllib/Sources/HDL Counter  CountType=Count limited  CountInit=0  CountStep=1  CountMax=6  CountFromType=Initial value  CountFrom=0  CountResetPort=on  CountLoadPort=off  CountEnbPort=on  CountDirPort=off  CountHitOutputPort=off  CountDataType=Unsigned  CountWordLen=8  CountFracLen=0  CountSampTime=1
  IsNonZero : simulink/Logic and Bit Operations/Compare To Zero  relop=~=  OutDataTypeStr=boolean
      settings: LibrarySourceBlock=|
      | simulink/Quick Insert/Logic and Bit
      | Operations/IsNonZero
  IsZero : simulink/Logic and Bit Operations/Compare To Zero  relop===  OutDataTypeStr=boolean
      settings: LibrarySourceBlock=|
      | simulink/Quick Insert/Logic and Bit
      | Operations/IsZero
  Logical Operator : Logic  AllPortsSameDT=off  OutDataTypeStr=boolean
  Logical Operator1 : Logic  AllPortsSameDT=off  OutDataTypeStr=boolean
  Logical Operator2 : Logic  Operator=OR  AllPortsSameDT=off  OutDataTypeStr=boolean
  NOT : Logic  Operator=NOT  IconShape=distinctive  AllPortsSameDT=off  OutDataTypeStr=boolean
  NOT1 : Logic  Operator=NOT  IconShape=distinctive  AllPortsSameDT=off  OutDataTypeStr=boolean
  MODCOD bit : Outport
  validOut : Outport  Port=2
  startOfBits : Outport  Port=3
  wires:
  IsZero/1 -> Logical Operator1/2, Logical Operator/1
  HDL Counter1/1 -> MODCOD bit/1, IsNonZero/1, IsZero/1
  Trigger/1 -> NOT/1
  Data Type Conversion/1 -> HDL Counter1/2
  Constant/1 -> Data Type Conversion/1
  NOT/1 -> Logical Operator/2
  Logical Operator/1 -> NOT1/1, HDL Counter1/1
  NOT1/1 -> Logical Operator1/1
  Logical Operator1/1 -> Logical Operator2/1, startOfBits/1
  IsNonZero/1 -> Logical Operator2/2
  Logical Operator2/1 -> validOut/1

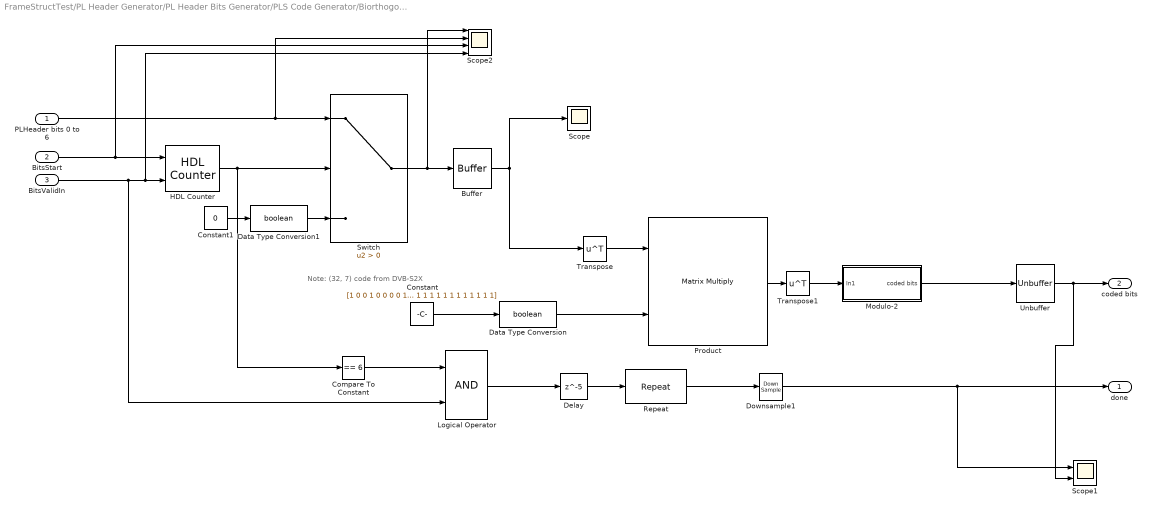
== system FrameStructTest/PL Header Generator/PL Header Bits Generator/PLS Code Generator/Biorthogonal code ==
  note: Note: (32, 7) code from DVB-S2X
  PLHeader bits 0 to 6 : Inport
  BitsStart : Inport  Port=2
  BitsValidIn : Inport  Port=3
  Buffer : Buffer  N=7  OutputFrames=off
  Compare To Constant : simulink/Logic and Bit Operations/Compare To Constant  relop===  const=6  OutDataTypeStr=boolean
  Constant : Constant  Value=[1 0 0 1 0 0 0 0 1 0 1 0 1 1 0 0 0 0 1 0 1 1 0 1 1 1 0 1 1 1 0 1; 0 1 0 1 0 1 0 1 0 1 0 1 0 1 0 1 0 1 0 1 0 1 0 1 0 1 0 1 0 1 0 1; 0 0 1 1 0 0 1 1 0 0 1 1 0 0 1 1 0 0 1 1 0 0 1 1 0 0 1 1 0 0 1 1; 0 0 0 0 1 1 1 1 0 0 0 0 1 1 1 1 0 0 0 0 1 1 1 1 0 0 0 0 1 1 1 1; 0 0 0 0 0 0 0 0 1 1 1 1 1 1 1 1 0 0 0 0 0 0 0 0 1 1 1 1 1 1 1 1; 0 0 0 0 0 0 0 0 0 0 0 0 0 0 0 0 1 1 1 1 1 1 1 1 1 1 1 1 1 1 1 1; 1 1 1 1 1 1 1 1 1 1 1 1 1 1 1 1 1 1 1 1 1 1 1 1 1 1 1 1 1 1 1 1]  VectorParams1D=off  OutDataTypeStr=boolean  SampleTime=7*f_s  LockScale=on
  Constant1 : Constant  Value=0  SampleTime=f_s
  Data Type Conversion : DataTypeConversion  OutDataTypeStr=boolean  SaturateOnIntegerOverflow=off  RndMeth=Floor
  Data Type Conversion1 : DataTypeConversion  OutDataTypeStr=boolean  SaturateOnIntegerOverflow=off  RndMeth=Floor
  Delay : Delay  DelayLength=5
  Downsample1 : DownSample  N=7  RateOptions=Allow multirate processing
  HDL Counter : hdlsllib/Sources/HDL Counter  CountType=Count limited  CountInit=0  CountStep=6  CountMax=25  CountFromType=Initial value  CountFrom=0  CountResetPort=on  CountLoadPort=off  CountEnbPort=on  CountDirPort=off  CountHitOutputPort=off  CountDataType=Unsigned  CountWordLen=8  CountFracLen=0  CountSampTime=1
  Logical Operator : Logic  AllPortsSameDT=off  OutDataTypeStr=boolean
  Modulo-2 : Subsystem
  Product : Product  Multiplication=Matrix(*)
  Repeat : dspsigops/Repeat  N=32  InputProcessing=Columns as channels (frame based)  RateOptions=Allow multirate processing  ic=0  mode=Unused parameter value
      settings: LibrarySourceBlock=commsequence2/Repeat
  Scope : Scope
  Scope1 : Scope  NumInputPorts=2
  Scope2 : Scope  NumInputPorts=4
  Switch : Switch  Criteria=u2 > Threshold  SaturateOnIntegerOverflow=off  InputSameDT=off
  Transpose : Math  Operator=transpose
  Transpose1 : Math  Operator=transpose
  Unbuffer : Unbuffer
  done : Outport
  coded bits : Outport  Port=2
  wires:
  Modulo-2/1(coded bits) -> Unbuffer/1
  Transpose/1 -> Product/1
  Constant/1 -> Data Type Conversion/1
  Buffer/1 -> Scope/1, Transpose/1
  Data Type Conversion/1 -> Product/2
  Product/1 -> Transpose1/1
  Constant1/1 -> Data Type Conversion1/1
  Data Type Conversion1/1 -> Switch/3
  BitsStart/1 -> Scope2/3, HDL Counter/1
  BitsValidIn/1 -> Logical Operator/2, Scope2/4, HDL Counter/2
  Switch/1 -> Scope2/1, Buffer/1
  PLHeader bits 0 to 6/1 -> Scope2/2, Switch/1
  Compare To Constant/1 -> Logical Operator/1
  Logical Operator/1 -> Delay/1
  Transpose1/1 -> Modulo-2/1(In1)
  Unbuffer/1 -> Scope1/2, coded bits/1
  HDL Counter/1 -> Compare To Constant/1, Switch/2
  Repeat/1 -> Downsample1/1
  Delay/1 -> Repeat/1
  Downsample1/1 -> done/1, Scope1/1
